simulink model "car_model"  (R2017b)
settings: Solver=ode3  StartTime=0.0  StopTime=inf  FixedStep=0.01  RelTol=1e-3  EnableMultiTasking=on
model workspace (MAT data in the model file):
  A = Simulink.Parameter
  A.Value = 2.4
  A.DataType = 'auto'
  A.Dimensions = [1 1]
  Cd = Simulink.Parameter
  Cd.Value = 0.32
  Cd.DataType = 'auto'
  Cd.Dimensions = [1 1]
  Cr = Simulink.Parameter
  Cr.Value = 0.01
  Cr.DataType = 'auto'
  Cr.Dimensions = [1 1]
  Tm = Simulink.Parameter
  Tm.Value = 190
  Tm.DataType = 'auto'
  Tm.Dimensions = [1 1]
  betac = Simulink.Parameter
  betac.Value = 0.4
  betac.DataType = 'auto'
  betac.Dimensions = [1 1]
  g = Simulink.Parameter
  g.Value = 9.8
  g.DataType = 'auto'
  g.Dimensions = [1 1]
  m = Simulink.Parameter
  m.Value = 1000
  m.DataType = 'auto'
  m.Dimensions = [1 1]
  omegam = Simulink.Parameter
  omegam.Value = 420
  omegam.DataType = 'auto'
  omegam.Dimensions = [1 1]
  rho = Simulink.Parameter
  rho.Value = 1.2
  rho.DataType = 'auto'
  rho.Dimensions = [1 1]
libraries: simulink x2, simulink_extras x1
settings Model: Creator=root  LastModifiedBy=Conor
settings SolverCC: ShapePreserveControl=EnableAll
settings DataIOCC: ReturnWorkspaceOutputs=on
settings OptimizationCC: DefaultUnderspecifiedDataType=single  EfficientFloat2IntCast=on  LifeSpan=inf
settings DebuggingCC: SFUnexpectedBacktrackingDiag=warning  SFNoUnconditionalDefaultTransitionDiag=warning  SFExecutionAtInitializationDiag=none
settings HardwareCC: ProdBitPerSizeT=32  ProdBitPerPtrDiffT=32  ProdWordSize=32  ProdHWDeviceType=Specified
settings ModelReferenceCC: PropagateSignalLabelsOutOfModel=off
settings CodeAppCC: StateflowObjectComments=on
settings GRTTargetCC: TargetLangStandard=C89/C90 (ANSI)  GeneratePreprocessorConditionals=Disable all
settings ConfigComp: CovMetricSettings=dw  CovHtmlReporting=on  CovSaveCumulativeToWorkspaceVar=on  CovSaveSingleToWorkspaceVar=on  CovExternalEMLEnable=off
settings SimscapeCC: SimscapeNormalizeSystem=off
settings ConfigurationSet: Description=SimMechanics 2G

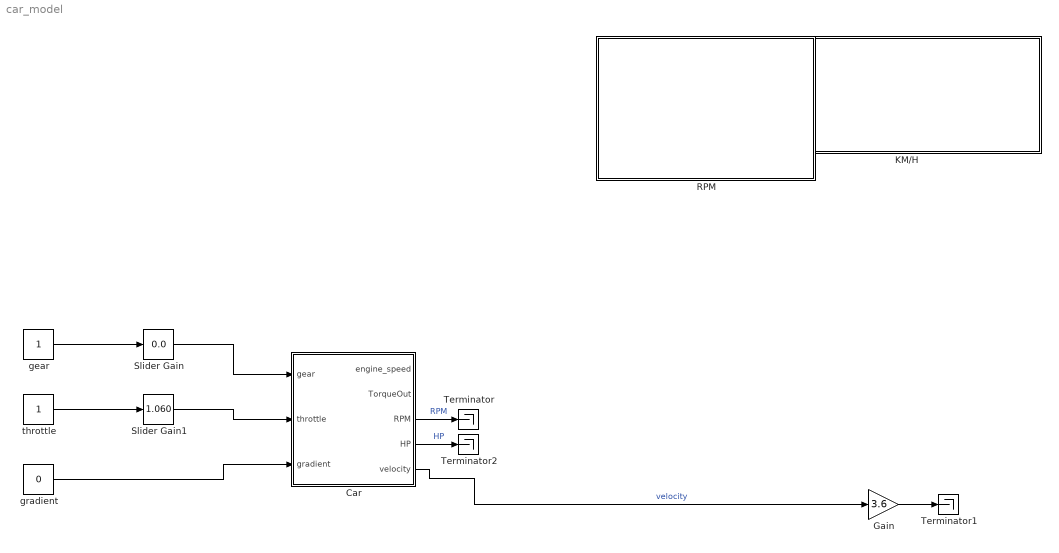
== system car_model ==
  Car : Subsystem
  Gain : Gain  Gain=3.6
  KM/H : Subsystem  DialogController=hmiCreateDDGDialog  IsWebBlock=on  mask(MathWorksWebBlock){webBlockId=13650363-325a-439c-a661-e207cee37534, webBlockType=semicirculargauge, ShowInLibBrowser=on, ShowInitialText=on, HMISrcModelName=car_model}
      mask prompts: webBlockId "WebBlock Id"; webBlockType "WebBlock Type"; HMISrcModelName "Source Model"
      mask Help: helpview([docroot '/mapfiles/simulink.map'], 'hmi_half_gauge')
      mask Display:
      | if strcmp(get_param(bdroot(gcb),'BlockDiagramType'), 'library')
      |     image([(matlabroot) '/toolbox/simulink/hmi/icons/SemicircularGauge.png']);
      | end
  RPM : Subsystem  DialogController=hmiCreateDDGDialog  IsWebBlock=on  mask(MathWorksWebBlock){webBlockId=7f42bb37-8e08-45c6-b6e3-9bc8244116c7, webBlockType=circulargauge, ShowInLibBrowser=on, ShowInitialText=on, HMISrcModelName=car_model}
      mask prompts: webBlockId "WebBlock Id"; webBlockType "WebBlock Type"; HMISrcModelName "Source Model"
      mask Help: helpview([docroot '/mapfiles/simulink.map'], 'hmi_gauge')
      mask Display:
      | if strcmp(get_param(bdroot(gcb),'BlockDiagramType'), 'library')
      |     image([(matlabroot) '/toolbox/simulink/hmi/icons/CircularGauge.png']);
      | end
  Slider Gain : simulink/Math Operations/Slider Gain  gain=0.0  low=0  high=5
  Slider Gain1 : simulink/Math Operations/Slider Gain  gain=1.060  low=-0.05  high=1.06
  Terminator : Terminator
  Terminator1 : Terminator
  Terminator2 : Terminator
  gear : Constant
  gradient : Constant  Value=0
  throttle : Constant
  wires:
  Car/5(velocity) -> Gain/1  "velocity"
  Car/3(RPM) -> Terminator/1  "RPM"
  Gain/1 -> Terminator1/1
  Car/4(HP) -> Terminator2/1  "HP"
  gradient/1 -> Car/3(gradient)
  gear/1 -> Slider Gain/1
  Slider Gain/1 -> Car/1(gear)
  throttle/1 -> Slider Gain1/1
  Slider Gain1/1 -> Car/2(throttle)

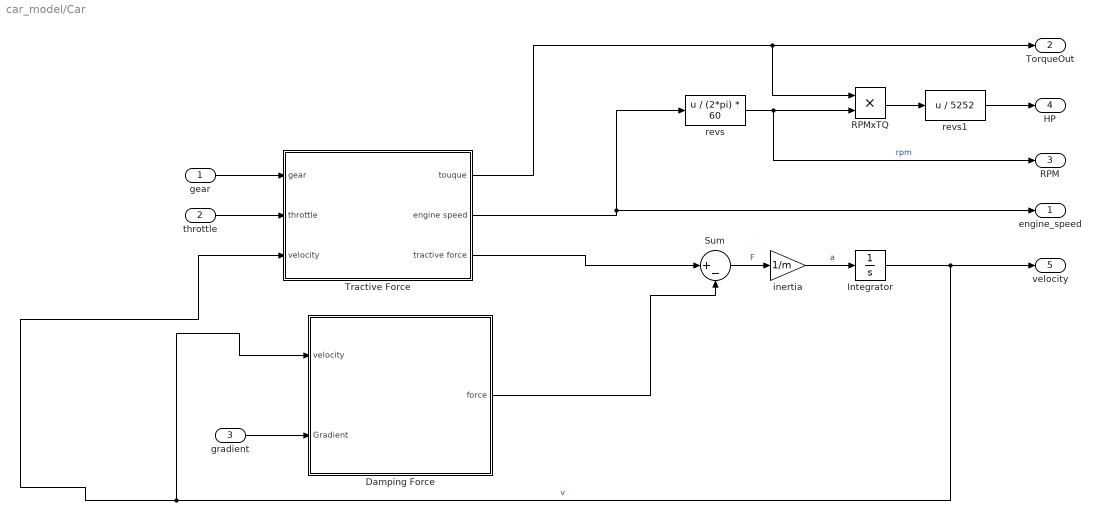
== system car_model/Car ==
  gear : Inport
  throttle : Inport  Port=2  OutMin=0  OutMax=1
  gradient : Inport  Port=3
  Damping Force : Subsystem
  Integrator : Integrator
  RPMxTQ : Product
  Sum : Sum  Inputs=|+-
  Tractive Force : Subsystem
  inertia : Gain  Gain=1/m
  revs : Fcn  Expr=u / (2*pi) * 60
  revs1 : Fcn  Expr=u / 5252
  engine_speed : Outport
  TorqueOut : Outport  Port=2
  RPM : Outport  Port=3
  HP : Outport  Port=4
  velocity : Outport  Port=5
  wires:
  inertia/1 -> Integrator/1  "a"
  Sum/1 -> inertia/1  "F"
  Integrator/1 -> Tractive Force/3(velocity), Damping Force/1(velocity), velocity/1  "v"
  revs/1 -> RPM/1, RPMxTQ/2  "rpm"
  RPMxTQ/1 -> revs1/1
  revs1/1 -> HP/1
  Tractive Force/2(engine speed) -> revs/1, engine_speed/1
  Tractive Force/1(touque) -> TorqueOut/1, RPMxTQ/1
  gear/1 -> Tractive Force/1(gear)
  throttle/1 -> Tractive Force/2(throttle)
  Tractive Force/3(tractive force) -> Sum/1
  gradient/1 -> Damping Force/2(Gradient)
  Damping Force/1(force) -> Sum/2

== system car_model/KM//H ==

== system car_model/RPM ==

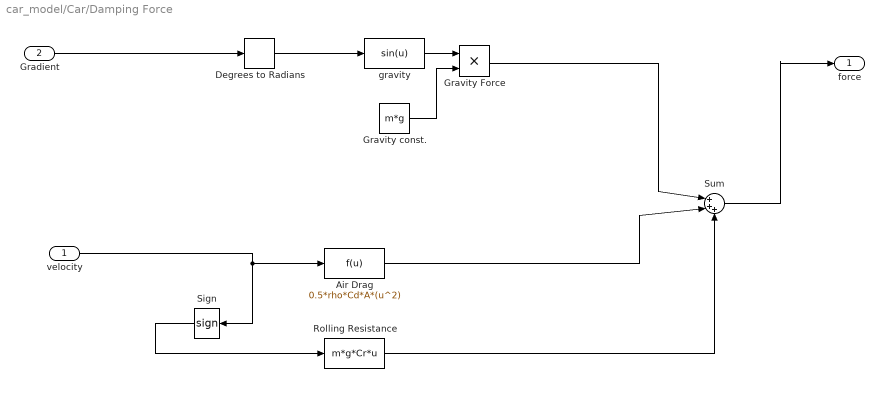
== system car_model/Car/Damping Force ==
  velocity : Inport
  Gradient : Inport  Port=2
  Air Drag : Fcn  Expr=0.5*rho*Cd*A*(u^2)
  Degrees to Radians : simulink_extras/Transformations/Degrees to Radians
  Gravity Force : Product
  Gravity const. : Constant  Value=m*g
  Rolling Resistance : Fcn  Expr=m*g*Cr*u
  Sign : Signum
  Sum : Sum  Inputs=|+++
  gravity : Fcn  Expr=sin(u)
  force : Outport
  wires:
  Sign/1 -> Rolling Resistance/1
  Rolling Resistance/1 -> Sum/3
  Gravity const./1 -> Gravity Force/2
  Gradient/1 -> Degrees to Radians/1
  Degrees to Radians/1 -> gravity/1
  gravity/1 -> Gravity Force/1
  Air Drag/1 -> Sum/2
  Gravity Force/1 -> Sum/1
  velocity/1 -> Air Drag/1, Sign/1
  Sum/1 -> force/1

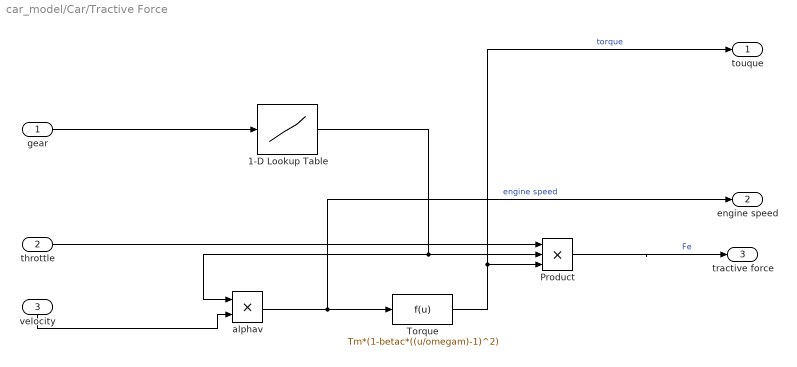
== system car_model/Car/Tractive Force ==
  gear : Inport
  throttle : Inport  Port=2
  velocity : Inport  Port=3
  1-D Lookup Table : Lookup_n-D  NumberOfTableDimensions=1  BreakpointsForDimension1=int16([1,2,3,4,5]);  Table=int16([40,25,16,12,10]);  InternalRulePriority=Speed  RndMeth=Simplest  InputSameDT=on
  Product : Product  Inputs=3
  Torque : Fcn  Expr=Tm*(1-betac*((u/omegam)-1)^2)
  alphav : Product
  touque : Outport
  engine speed : Outport  Port=2
  tractive force : Outport  Port=3
  wires:
  gear/1 -> 1-D Lookup Table/1
  Torque/1 -> touque/1, Product/3  "torque"
  throttle/1 -> Product/1
  1-D Lookup Table/1 -> Product/2, alphav/1
  alphav/1 -> engine speed/1, Torque/1  "engine speed"
  Product/1 -> tractive force/1  "Fe"
  velocity/1 -> alphav/2
